simulink model "pathfollowing"  (R2022b)
settings: Solver=VariableStepAuto  StartTime=0.0  StopTime=10.0  RelTol=1e-3
settings Model: Creator=XinyiWu  LastModifiedBy=XinyiWu

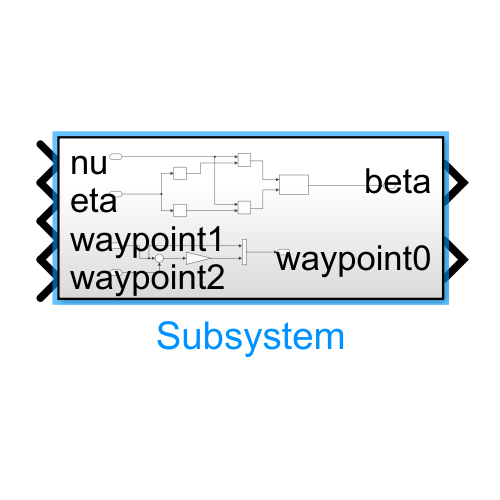
[thumbnail: Simulink's stored preview of the top-level diagram]
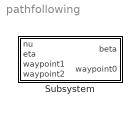
== system pathfollowing ==
  Subsystem : Subsystem

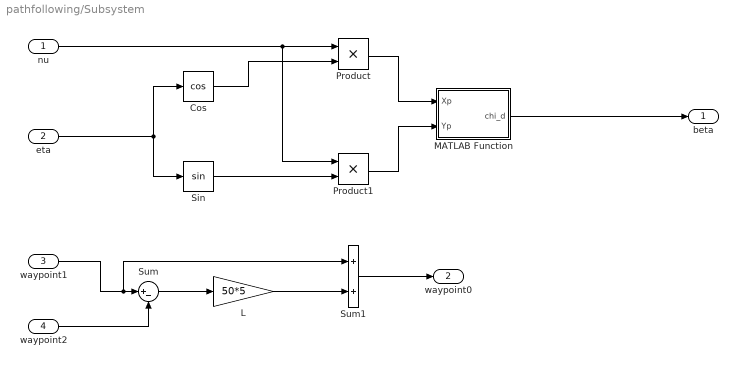
== system pathfollowing/Subsystem ==
  nu : Inport
  eta : Inport  Port=2
  waypoint1 : Inport  Port=3
  waypoint2 : Inport  Port=4
  Cos : Trigonometry  Operator=cos
  L : Gain  Gain=50*5
  MATLAB Function : MATLAB Function  TreatAsAtomicUnit=on
  Product : Product
  Product1 : Product
  Sin : Trigonometry
  Sum : Sum  Inputs=|+-
  Sum1 : Sum
  beta : Outport
  waypoint0 : Outport  Port=2
  wires:
  eta/1 -> Sin/1, Cos/1
  nu/1 -> Product1/1, Product/1
  Cos/1 -> Product/2
  Sin/1 -> Product1/2
  Product/1 -> MATLAB Function/1(Xp)
  Product1/1 -> MATLAB Function/2(Yp)
  MATLAB Function/1(chi_d) -> beta/1
  waypoint1/1 -> Sum1/1, Sum/1
  waypoint2/1 -> Sum/2
  Sum/1 -> L/1
  L/1 -> Sum1/2
  Sum1/1 -> waypoint0/1

== matlab function pathfollowing/Subsystem/MATLAB Function ==
  data: Xp input; chi_d output; Yp input
function chi_d = fcn(Xp,Yp)

chi_d = atan2(Xp,Yp);
